simulink model "ex5_3"  (R2020a)
settings: Solver=VariableStepAuto  StartTime=0.0  StopTime=10.0  RelTol=1e-3
settings Model: Creator=반달  LastModifiedBy=반달

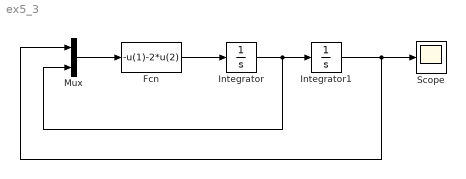
== system ex5_3 ==
  Fcn : Fcn  Expr=-u(1)-2*u(2)
  Integrator : Integrator
  Integrator1 : Integrator  InitialCondition=2
  Mux : Mux  Inputs=2
  Scope : Scope
  wires:
  Integrator/1 -> Mux/2, Integrator1/1
  Mux/1 -> Fcn/1
  Fcn/1 -> Integrator/1
  Integrator1/1 -> Mux/1, Scope/1
